simulink model "lab1_dybac_L"  (R2023a)
settings: Solver=ode5  StartTime=0  StopTime=12  FixedStep=.005  MaxStep=0.02  RelTol=1e-3  AbsTol=1e-6
values from neighbouring files (symbols this model uses):
  A = [0 1 0 0 ; ((M+m)*g)/(M*L) 0 0 0; 0 0 0 1; (-m*g)/M 0 0 0]    [TP1.m]
  B = [0; -1/M*L;0;1/M]    [TP1.m]
  C = [1 0 0 0; 0 0 1 0]    [TP1.m]
  C_block = eye(4)    [TP1.m]
  D = [0;0;0;0]    [TP1.m]
  F = -place(A,B,p_desired)    [TP1.m]
  K_fast = place(A.',C.',p_fast).'    [TP1.m]
  x_0 = [0.1;0;0.1;0]    [TP1.m]
settings Model: Creator=user  LastModifiedBy=jlancha2023
settings SolverCC: AutoScaleAbsTol=off  AlgebraicLoopSolver=TrustRegion
settings DataIOCC: ExternalInput=[]  InitialState=[]  SaveFormat=Array  SignalLoggingSaveFormat=ModelDataLogs  SaveOutput=off  SaveTime=off  ReturnWorkspaceOutputs=off
settings OptimizationCC: BooleanDataType=off  ExpressionDepthLimit=2147483647  InitFltsAndDblsToZero=on  LifeSpan=inf
settings DebuggingCC: SaveWithParameterizedLinksMsg=none  UnderspecifiedInitializationDetection=Classic  MergeDetectMultiDrivingBlocksExec=none  SignalResolutionControl=TryResolveAllWithWarning  MultiTaskDSMMsg=warning  MultiTaskCondExecSysMsg=none  FcnCallInpInsideContextMsg=warning  UnconnectedInputMsg=warning  UnconnectedOutputMsg=warning  UnconnectedLineMsg=warning  StateNameClashWarn=warning  SFUnexpectedBacktrackingDiag=warning  SFNoUnconditionalDefaultTransitionDiag=warning  SFExecutionAtInitializationDiag=none  ArithmeticOperatorsInVariantConditions=warning
settings HardwareCC: ProdBitPerPointer=32  ProdBitPerSizeT=32  ProdBitPerPtrDiffT=32  ProdLargestAtomicFloat=None  ProdIntDivRoundTo=Undefined  ProdEndianess=Unspecified  ProdWordSize=32  ProdHWDeviceType=32-bit Generic  TargetUnknown=on
settings ModelReferenceCC: EnableRefExpFcnMdlSchedulingChecks=on  PropagateSignalLabelsOutOfModel=off
settings SFSimCC: SimUseLocalCustomCode=off  CustomCodeUndefinedFunction=UseInterfaceOnly
settings RTWCC: RTWUseLocalCustomCode=off
settings CodeAppCC: StateflowObjectComments=on
settings GRTTargetCC: TargetFcnLib=ansi_tfl_tmw.mat  TargetLangStandard=C89/C90 (ANSI)  CombineOutputUpdateFcns=off  GRTInterface=on
settings ConfigComp: CovMetricSettings=dw  CovSaveCumulativeToWorkspaceVar=on  CovSaveSingleToWorkspaceVar=on  CovExternalEMLEnable=off

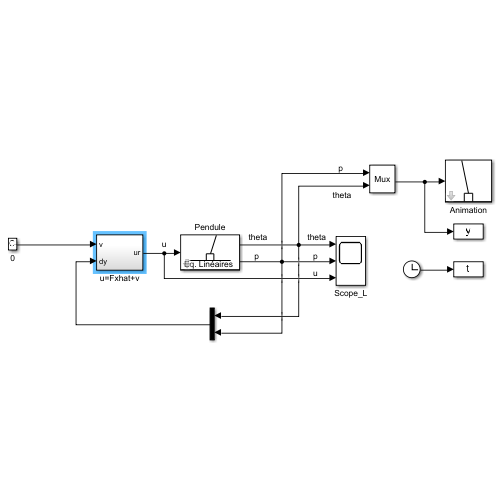
[thumbnail: Simulink's stored preview of the top-level diagram]
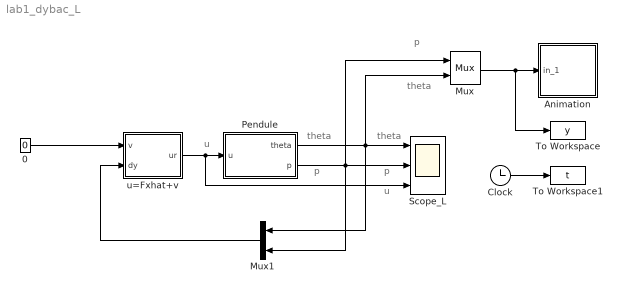
== system lab1_dybac_L ==
  note: p
  note: theta
  note: p
  note: theta
  note: theta
  note: p
  note: u
  note: u
  0 : Constant  Value=0
  Animation : Subsystem  mask(Animation du déplacement du pendule inverse){}
      mask Help: Fonction d'animation du pendule inverse (voir s_fonction tp_pendan_g.m.
      mask Display: plot([-10 10],[0 0],[-2 -2 2 2],[0 1 1 0],[0 -3],[1 5])
  Clock : Clock
  Mux : Mux  Inputs=2
  Mux1 : Mux  Inputs=2
  Pendule : Subsystem  mask(Pendule inverse sur un chariot (éq. Linéaires).){A=A, B=B, C=C, D=D, x0=[0.1 0 0.1 0]}
      mask prompts: x0 "Conditions initiales"
      mask help: Utiliser le menu "Look under mask" pour voir les équations linéarisées de la dynamique (celles de l'énoncé du TP)
      mask Help: Description Linéarisée de la dynamique d'un pendule inverse sur un chariot.
      mask Display:
      | plot([-10 10],[1 1],[-2 -2 2 2],[1 2 2 1],[0 3],[2 5])
      | text(-12,0.5,'Eq. Linéaires')
      | plot([-14 14],[-0.5 -0.5])
  Scope_L : Scope  NumInputPorts=3
  To Workspace : ToWorkspace  VariableName=y  SampleTime=0.1
  To Workspace1 : ToWorkspace  VariableName=t  SampleTime=0.1
  u=Fxhat+v : Subsystem
  wires:
  Mux/1 -> To Workspace/1, Animation/1(in_1)
  Clock/1 -> To Workspace1/1
  u=Fxhat+v/1(ur) -> Pendule/1(u), Scope_L/3
  Pendule/2(p) -> Mux1/2, Scope_L/2, Mux/1
  Pendule/1(theta) -> Mux1/1, Scope_L/1, Mux/2
  Mux1/1 -> u=Fxhat+v/2(dy)
  0/1 -> u=Fxhat+v/1(v)

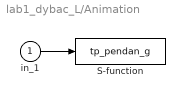
== system lab1_dybac_L/Animation ==
  in_1 : Inport
  S-function : S-Function  FunctionName=tp_pendan_g  SFunctionDeploymentMode=off  EnableBusSupport=off
      settings: DeleteFcn=pendan([],[],[],'DeleteBlock');
  wires:
  in_1/1 -> S-function/1

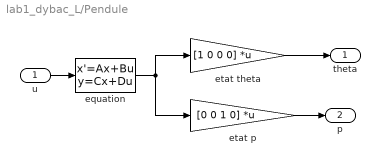
== system lab1_dybac_L/Pendule ==
  u : Inport
  equation : StateSpace  A=A  B=B  C=eye(4)  D=zeros(4,1)  InitialCondition=x0
  etat p : Gain  Gain=[0 0 1 0]  Multiplication=Matrix(K*u)  SaturateOnIntegerOverflow=on  OutDataTypeStr=Inherit: Same as input  ParamDataTypeStr=Inherit: Same as input
  etat theta : Gain  Gain=[1 0 0 0]  Multiplication=Matrix(K*u)  SaturateOnIntegerOverflow=on  OutDataTypeStr=Inherit: Same as input  ParamDataTypeStr=Inherit: Same as input
  theta : Outport
  p : Outport  Port=2
  wires:
  equation/1 -> etat p/1, etat theta/1
  etat p/1 -> p/1
  u/1 -> equation/1
  etat theta/1 -> theta/1

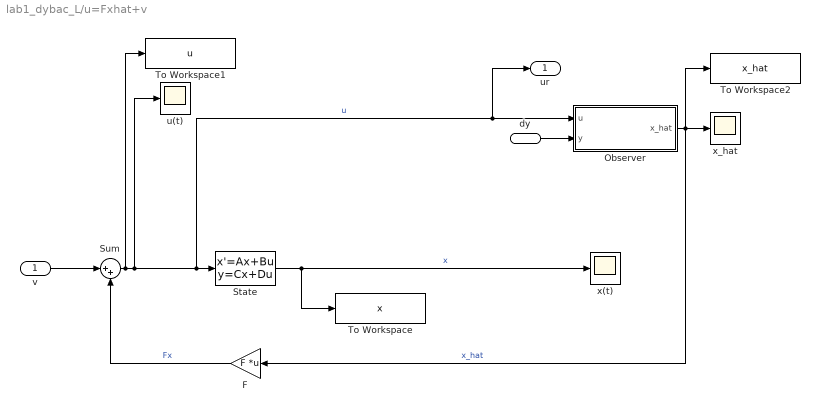
== system lab1_dybac_L/u=Fxhat+v ==
  v : Inport
  dy : Inport  Port=2
  F : Gain  Gain=F  Multiplication=Matrix(K*u)
  Observer : Subsystem
  State : StateSpace  A=A  B=B  C=C_block  D=D  InitialCondition=x_0
  Sum : Sum  Inputs=|++
  To Workspace : ToWorkspace  VariableName=x  SampleTime=-1
  To Workspace1 : ToWorkspace  VariableName=u  SampleTime=-1
  To Workspace2 : ToWorkspace  VariableName=x_hat  SaveFormat=Timeseries  SampleTime=-1
  u(t) : Scope
  x(t) : Scope
  x_hat : Scope
  ur : Outport
  wires:
  v/1 -> Sum/1
  Sum/1 -> ur/1, Observer/1(u), State/1, u(t)/1, To Workspace1/1  "u"
  F/1 -> Sum/2  "Fx"
  Observer/1(x_hat) -> To Workspace2/1, F/1, x_hat/1  "x_hat"
  State/1 -> x(t)/1, To Workspace/1  "x"
  dy/1 -> Observer/2(y)

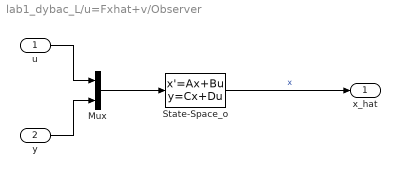
== system lab1_dybac_L/u=Fxhat+v/Observer ==
  u : Inport
  y : Inport  Port=2
  Mux : Mux  Inputs=2
  State-Space_o : StateSpace  A=A - K_fast*C  B=[B K_fast]  C=C_block  D=zeros(4,3)  InitialCondition=[0;0;0;0]
  x_hat : Outport
  wires:
  u/1 -> Mux/1
  y/1 -> Mux/2
  Mux/1 -> State-Space_o/1
  State-Space_o/1 -> x_hat/1  "x"
